simulink model "lab_1_5"  (R2019a)
settings: Solver=VariableStepAuto  StartTime=0.0  StopTime=10.0  RelTol=1e-3
settings Model: Creator=ADMIN  LastModifiedBy=ADMIN

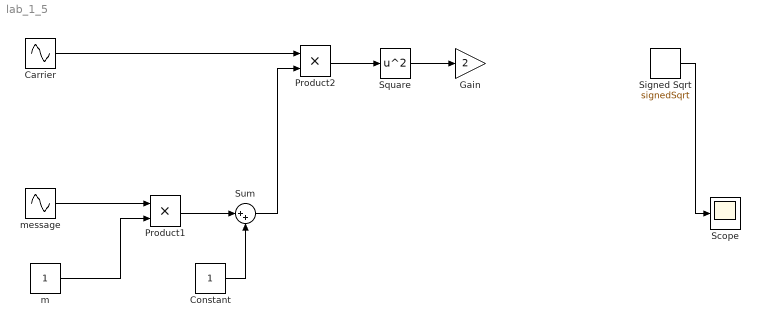
== system lab_1_5 ==
  Carrier : Sin  Frequency=2*pi*25  SampleTime=1/5000
  Constant : Constant
  Gain : Gain  Gain=2
  Product1 : Product
  Product2 : Product
  Scope : Scope
  Signed Sqrt : Sqrt  Operator=signedSqrt  SaturateOnIntegerOverflow=on
  Square : Math  Operator=square  SaturateOnIntegerOverflow=on
  Sum : Sum  Inputs=|++
  "m " : Constant
  "message " : Sin  Bias=2*pi  SampleTime=1/5000
  wires:
  Constant/1 -> Sum/2
  Sum/1 -> Product2/2
  Product1/1 -> Sum/1
  "message "/1 -> Product1/1
  Carrier/1 -> Product2/1
  "m "/1 -> Product1/2
  Product2/1 -> Square/1
  Square/1 -> Gain/1
  Signed Sqrt/1 -> Scope/1
